simulink model "StarMac_Model"  (Simulink 7.1)
settings: Solver=FixedStepDiscrete  StartTime=0.0  StopTime=10.0  RelTol=1e-3
undefined symbols (not defined in the file or in its folder): schedule, ToverTh
libraries: simulink x10, truetime x2, aero_sim_lib x1
settings Model: Creator=jporter  LastModifiedBy=jporter

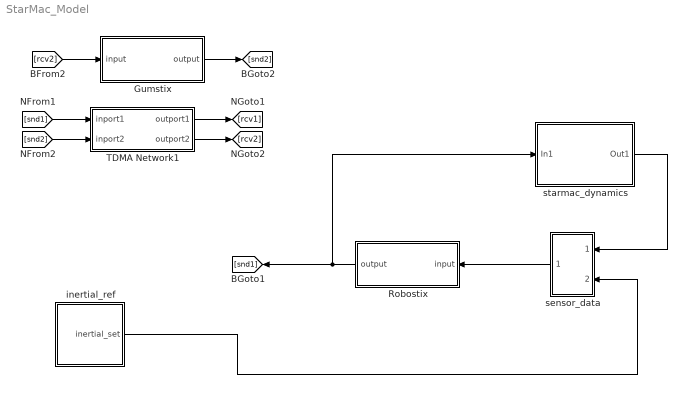
== system StarMac_Model ==
  Gumstix : Subsystem
  Robostix : Subsystem  Orientation=left
  TDMA Network1 : Subsystem
  inertial_ref : Subsystem
  sensor_data : Subsystem  Orientation=left
  starmac_dynamics : Subsystem
  wires:
  inertial_ref/1(inertial_set) -> sensor_data/2(In2)
  starmac_dynamics/1(Out1) -> sensor_data/1(In1)
  TDMA Network1/1(outport1) -> [rcv1]
  [snd1] -> TDMA Network1/1(inport1)
  TDMA Network1/2(outport2) -> [rcv2]
  [snd2] -> TDMA Network1/2(inport2)
  Robostix/1(output) -> [snd1], starmac_dynamics/1(In1)
  [rcv2] -> Gumstix/1(input)
  Gumstix/1(output) -> [snd2]
  sensor_data/1(Out1) -> Robostix/1(input)

== system StarMac_Model/Gumstix ==
  input : Inport
  Ground1 : Ground
  Gumstix_Output : Scope
      settings: DataFormat=Array
  Gumstix_Schedule : Scope
      settings: DataFormat=Array
  Terminator1 : Terminator
  Terminator2 : Terminator
  Terminator3 : Terminator
  TrueTime Kernel : Subsystem  mask{sfun=Generic_Init, args=schedule, clockdrift=0, clockoffset=0}
      mask prompts: sfun "Name of init function (MEX or MATLAB)"; args "Init function argument"; clockdrift "Clock drift"; clockoffset "Clock offset"
  output : Outport
  wires:
  input/1 -> TrueTime Kernel/3(Rcv)
  Ground1/1 -> TrueTime Kernel/1(A/D), TrueTime Kernel/2(Interrupts)
  TrueTime Kernel/2(Snd) -> output/1, Gumstix_Output/1
  TrueTime Kernel/1(D/A) -> Terminator1/1
  TrueTime Kernel/3(Schedule) -> Gumstix_Schedule/1
  TrueTime Kernel/4(Monitors) -> Terminator2/1
  TrueTime Kernel/5(P) -> Terminator3/1

== system StarMac_Model/Robostix ==
  input : Inport
  Ground1 : Ground
  Robostix_Output : Scope
      settings: DataFormat=Array
  Robostix_Schedule : Scope
      settings: DataFormat=Array
  Terminator1 : Terminator
  Terminator2 : Terminator
  Terminator3 : Terminator
  TrueTime Kernel : Subsystem  mask{sfun=Generic_Init, args=schedule, clockdrift=0, clockoffset=0}
      mask prompts: sfun "Name of init function (MEX or MATLAB)"; args "Init function argument"; clockdrift "Clock drift"; clockoffset "Clock offset"
  output : Outport
  wires:
  input/1 -> TrueTime Kernel/3(Rcv)
  Ground1/1 -> TrueTime Kernel/1(A/D), TrueTime Kernel/2(Interrupts)
  TrueTime Kernel/2(Snd) -> output/1, Robostix_Output/1
  TrueTime Kernel/1(D/A) -> Terminator1/1
  TrueTime Kernel/3(Schedule) -> Robostix_Schedule/1
  TrueTime Kernel/4(Monitors) -> Terminator2/1
  TrueTime Kernel/5(P) -> Terminator3/1

== system StarMac_Model/TDMA Network1 ==
  inport1 : Inport
  inport2 : Inport  Port=2
  Demux1 : Demux  Outputs=2
  Mux1 : Mux  Inputs=2
  Network_Schedule : Scope
      settings: DataFormat=Array
  TrueTime Network : Subsystem  mask{nwtype=TDMA, nwnbr=1, nnodes=2, rate=100000, minsize=4096, lossprob=0, bandwidths=[0.5 0.5], slotsize=4096, schedule=[1 2], memsize=671088640, buftype=Common Buffer, overflow=Retransmit}
      mask prompts: nwtype "Network type"; nwnbr "Network number"; nnodes "Number of nodes"; rate "Data rate (bits/s)"; minsize "Minimum frame size (bits)"; lossprob "Loss probability (0-1)"; bandwidths "Bandwidth allocations"; slotsize "Slotsize (bits)"; schedule "Cyclic schedule"; memsize "Total switch memory (bits)"; buftype "Switch buffer type"; overflow "Switch overflow behavior"
      mask StyleString: popup(CSMA/CD (Ethernet)|CSMA/AMP (CAN)|Round Robin|FDMA|TDMA|Switched Ethernet),edit,edit,edit,edit,edit,edit,edit,edit,edit,popup(Common buffer|Symmetric output buffers),popup(Retransmit|Drop)
  outport1 : Outport
  outport2 : Outport  Port=2
  wires:
  Mux1/1 -> TrueTime Network/1(Snd)
  TrueTime Network/1(Rcv) -> Demux1/1
  TrueTime Network/2(Schedule) -> Network_Schedule/1
  Demux1/1 -> outport1/1
  inport1/1 -> Mux1/1
  Demux1/2 -> outport2/1
  inport2/1 -> Mux1/2

== system StarMac_Model/inertial_ref ==
  Signal Generator : SignalGenerator  Amplitude=20*[1 -1 .5]  Frequency=.5*.0625*ones(3,1)
  inertial_set : Outport
  wires:
  Signal Generator/1 -> inertial_set/1

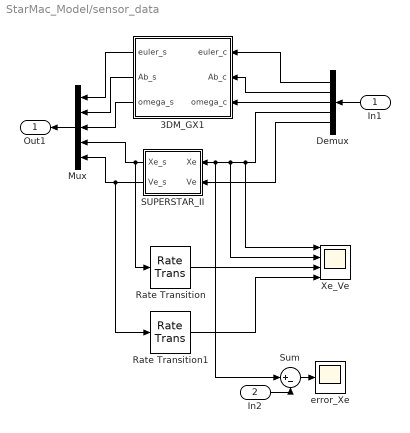
== system StarMac_Model/sensor_data ==
  In1 : Inport  Orientation=left
  In2 : Inport  Port=2
  3DM_GX1 : Subsystem  Orientation=left  mask{a_g_s=7000, g_max=5, g_g_s=8500, omega_max=300, Ts=.01}
      mask prompts: a_g_s "AccelGainScale:"; g_max "Max G (1 G = 9.81 m/s^2):"; g_g_s "GyroGainScale:"; omega_max "Mav Angular Velocity (deg/sec):"; Ts "Sample Rate (seconds):"
  Demux : Demux  Orientation=left  Outputs=5
  Mux : Mux  Orientation=left  Inputs=5
  Rate Transition : RateTransition
  Rate Transition1 : RateTransition
  SUPERSTAR_II : Subsystem  Orientation=left  mask{Ts=.2}
      mask prompts: Ts "Sample Rate (seconds):"
  Sum : Sum  Inputs=|+-  OutDataType=sfix(16)  OutScaling=2^0
  Xe_Ve : Scope  NumInputPorts=4
      settings: YMin=-5~-5~-5~-5  YMax=5~5~5~5
  error_Xe : Scope
  Out1 : Outport  Orientation=left
  wires:
  3DM_GX1/1(euler_s) -> Mux/1
  3DM_GX1/2(Ab_s) -> Mux/2
  3DM_GX1/3(omega_s) -> Mux/3
  SUPERSTAR_II/1(Xe_s) -> Mux/4, Rate Transition/1
  SUPERSTAR_II/2(Ve_s) -> Mux/5, Rate Transition1/1
  Demux/1 -> 3DM_GX1/1(euler_c)
  Demux/2 -> 3DM_GX1/2(Ab_c)
  Demux/3 -> 3DM_GX1/3(omega_c)
  Demux/4 -> Xe_Ve/1, Xe_Ve/2, SUPERSTAR_II/1(Xe), Sum/1
  Demux/5 -> SUPERSTAR_II/2(Ve)
  Rate Transition/1 -> Xe_Ve/3
  Rate Transition1/1 -> Xe_Ve/4
  Sum/1 -> error_Xe/1
  In1/1 -> Demux/1
  Mux/1 -> Out1/1
  In2/1 -> Sum/2

== system StarMac_Model/starmac_dynamics ==
  In1 : Inport
  Mux : Mux  Inputs=5
  Terminator : Terminator
  Terminator1 : Terminator
  starmac_dynamics : Subsystem  AncestorBlock=aero_sim_lib/starmac_dynamics  mask{M=1.8263, tau_motor=0.1, b=0.1, select_sub=Select Subsystem}
      mask prompts: M "UAV Mass (kg) [M]:"; tau_motor "Motor Time constant (s)[tau_motor]:"; b "Viscus Drag Coef. (N-s/m)[b]:"; select_sub "Select a model Subsystem:"
      mask StyleString: edit,edit,edit,popup(Select Subsystem|M:starmac_motor_dynamics|B:starmac_blade_flapping_effects|6:6DOF_Euler_Angles)
      mask CallbackString:
      | |||gcb_d=gcb;
      | mask_str = get_param(gcb_d, 'MaskValues');
      | if strcmp(mask_str{4}(1),'M')
      |     open_system([gcb_d '/starmac_motor_dynamics'],'mask');
      | elseif strcmp(mask_str{4}(1),'B')
      |     open_system([gcb_d '/starmac_blade_flapping_effects'],'mask');
      | elseif strcmp(mask_str{4}(1),'6')
      |     open_system([gcb_d '/6DOF_Euler_Angles'],'mask');
      | else
      |     return
      | end
      | set_param(gcb_d,'select_sub','Select Subsystem');
  wind_velocity : Constant  Value=zeros(3,1)  OutDataType=sfix(16)  OutScaling=2^0
  Out1 : Outport
  wires:
  wind_velocity/1 -> starmac_dynamics/2(wind_velocity)
  starmac_dynamics/1(Ve) -> Mux/1
  starmac_dynamics/2(Xe) -> Mux/2
  starmac_dynamics/4(DCM) -> Terminator/1
  starmac_dynamics/6(domega/dt) -> Terminator1/1
  Mux/1 -> Out1/1
  In1/1 -> starmac_dynamics/1(desired_motor_thrust)
  starmac_dynamics/3(euler) -> Mux/3
  starmac_dynamics/5(omega) -> Mux/4
  starmac_dynamics/7(Ab) -> Mux/5

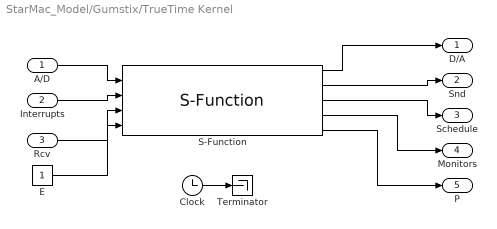
== system StarMac_Model/Gumstix/TrueTime Kernel ==
  A/D : Inport
  Interrupts : Inport  Port=2
  Rcv : Inport  Port=3
  Clock : Clock
      settings: Decimation=10
  E : Constant
  S-Function : truetime/TrueTime Kernel/S-Function
  Terminator : Terminator
  D/A : Outport
  Snd : Outport  Port=2
  Schedule : Outport  Port=3
  Monitors : Outport  Port=4
  P : Outport  Port=5
  wires:
  S-Function/5 -> P/1
  E/1 -> S-Function/4
  A/D/1 -> S-Function/1
  S-Function/2 -> Snd/1
  S-Function/1 -> D/A/1
  S-Function/3 -> Schedule/1
  S-Function/4 -> Monitors/1
  Interrupts/1 -> S-Function/2
  Rcv/1 -> S-Function/3
  Clock/1 -> Terminator/1

== system StarMac_Model/Robostix/TrueTime Kernel ==
  A/D : Inport
  Interrupts : Inport  Port=2
  Rcv : Inport  Port=3
  Clock : Clock
      settings: Decimation=10
  E : Constant
  S-Function : truetime/TrueTime Kernel/S-Function
  Terminator : Terminator
  D/A : Outport
  Snd : Outport  Port=2
  Schedule : Outport  Port=3
  Monitors : Outport  Port=4
  P : Outport  Port=5
  wires:
  S-Function/5 -> P/1
  E/1 -> S-Function/4
  A/D/1 -> S-Function/1
  S-Function/2 -> Snd/1
  S-Function/1 -> D/A/1
  S-Function/3 -> Schedule/1
  S-Function/4 -> Monitors/1
  Interrupts/1 -> S-Function/2
  Rcv/1 -> S-Function/3
  Clock/1 -> Terminator/1

== system StarMac_Model/TDMA Network1/TrueTime Network ==
  Snd : Inport
  ttnetwork : S-Function  FunctionName=ttnetwork  Parameters=nwtype,nwnbr,nnodes,rate,minsize,lossprob,bandwidths,slotsize,schedule,memsize,buftype,overflow  EnableBusSupport=off
  Rcv : Outport
  Schedule : Outport  Port=2
  wires:
  ttnetwork/2 -> Schedule/1
  ttnetwork/1 -> Rcv/1
  Snd/1 -> ttnetwork/1

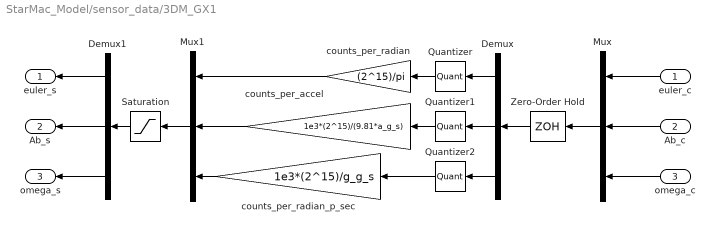
== system StarMac_Model/sensor_data/3DM_GX1 ==
  euler_c : Inport  Orientation=left
  Ab_c : Inport  Orientation=left  Port=2
  omega_c : Inport  Orientation=left  Port=3
  Demux : Demux  Orientation=left  Outputs=[3 3 3]
  Demux1 : Demux  Orientation=left  Outputs=[3 3 3]
  Mux : Mux  Orientation=left  Inputs=[3 3 3]
  Mux1 : Mux  Orientation=left  Inputs=3
  Quantizer : Quantizer  Orientation=left  QuantizationInterval=pi/(2^15)*ones(3,1)
  Quantizer1 : Quantizer  Orientation=left  QuantizationInterval=g_max*9.81/(2^15)*ones(3,1)
  Quantizer2 : Quantizer  Orientation=left  QuantizationInterval=(pi*omega_max/180)/(2^15)*ones(3,1)
  Saturation : Saturate  Orientation=left  UpperLimit=((2^15)-1)*ones(3*3,1)  LowerLimit=-(2^15)*ones(3*3,1)  OutDataType=sfix(16)  OutScaling=2^0
  Zero-Order Hold : ZeroOrderHold  Orientation=left  SampleTime=Ts
  counts_per_accel : Gain  Orientation=left  Gain=1e3*(2^15)/(9.81*a_g_s)  ParameterDataType=sfix(16)  ParameterScaling=2^0  OutDataType=sfix(16)  OutScaling=2^0
  counts_per_radian : Gain  Orientation=left  Gain=(2^15)/pi  ParameterDataType=sfix(16)  ParameterScaling=2^0  OutDataType=sfix(16)  OutScaling=2^0
  counts_per_radian_p_sec : Gain  Orientation=left  Gain=1e3*(2^15)/g_g_s  ParameterDataType=sfix(16)  ParameterScaling=2^0  OutDataType=sfix(16)  OutScaling=2^0
  euler_s : Outport  Orientation=left
  Ab_s : Outport  Orientation=left  Port=2
  omega_s : Outport  Orientation=left  Port=3
  wires:
  Mux/1 -> Zero-Order Hold/1
  euler_c/1 -> Mux/1
  Ab_c/1 -> Mux/2
  omega_c/1 -> Mux/3
  Zero-Order Hold/1 -> Demux/1
  Demux/1 -> Quantizer/1
  Demux/2 -> Quantizer1/1
  Quantizer/1 -> counts_per_radian/1
  Quantizer1/1 -> counts_per_accel/1
  counts_per_accel/1 -> Mux1/2
  counts_per_radian/1 -> Mux1/1
  Demux/3 -> Quantizer2/1
  counts_per_radian_p_sec/1 -> Mux1/3
  Quantizer2/1 -> counts_per_radian_p_sec/1
  Mux1/1 -> Saturation/1
  Saturation/1 -> Demux1/1
  Demux1/1 -> euler_s/1
  Demux1/2 -> Ab_s/1
  Demux1/3 -> omega_s/1

== system StarMac_Model/sensor_data/SUPERSTAR_II ==
  Xe : Inport  Orientation=left
  Ve : Inport  Orientation=left  Port=2
  Demux : Demux  Orientation=left  Outputs=[3 3]
  Mux : Mux  Orientation=left  Inputs=[3 3]
  ZOH : ZeroOrderHold  Orientation=left  SampleTime=Ts
  Xe_s : Outport  Orientation=left
  Ve_s : Outport  Orientation=left  Port=2
  wires:
  ZOH/1 -> Demux/1
  Ve/1 -> Mux/2
  Xe/1 -> Mux/1
  Mux/1 -> ZOH/1
  Demux/1 -> Xe_s/1
  Demux/2 -> Ve_s/1

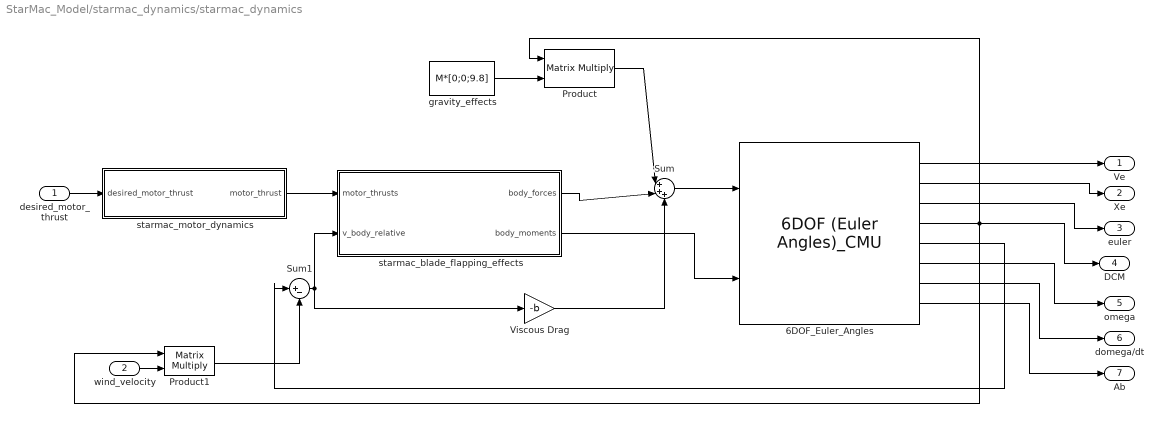
== system StarMac_Model/starmac_dynamics/starmac_dynamics ==
  desired_motor_thrust : Inport  OutDataType=sfix(16)  OutScaling=2^0
  wind_velocity : Inport  Port=2  OutDataType=sfix(16)  OutScaling=2^0
  6DOF_Euler_Angles : aero_sim_lib/6DOF (Euler Angles)_CMU  SystemSampleTime=-1  XYZe_0=[0.1;0.2;0]  Vb_0=[0;0;0]  euler_0=[0;0;0]  omega_0=[0;0;0]  M=M  I=diag([0.02759 0.02771 0.04806])
  Product : Product  Multiplication=Matrix(*)  OutDataType=sfix(16)  OutScaling=2^0  RndMeth=Zero
  Product1 : Product  Multiplication=Matrix(*)  OutDataType=sfix(16)  OutScaling=2^0  RndMeth=Zero
  Sum : Sum  Inputs=|+++  OutDataType=sfix(16)  OutScaling=2^0
  Sum1 : Sum  Inputs=|+-  OutDataType=sfix(16)  OutScaling=2^0
  Viscous Drag : Gain  Gain=-b  ParameterDataType=sfix(16)  ParameterScaling=2^0  OutDataType=sfix(16)  OutScaling=2^0
  gravity_effects : Constant  Value=M*[0;0;9.8]  OutDataType=sfix(16)  OutScaling=2^0
  starmac_blade_flapping_effects : Subsystem  AncestorBlock=aero_sim_lib/starmac_blade_flapping_effects  mask{select_sub=Select Subsystem}
      mask prompts: select_sub "Select Subsystem:"
      mask help:
      | Allows user to set parameters of various subsystems
      | within the Blade Flapping Effects Model
      mask Help:
      | Select a Subsystem To Set Various
      | Sub System Parameters
      mask StyleString: popup(Select Subsystem|V:starmac_vertical_effect_dynamics|B:starmac_body_moments|F:starmac_flapping_dynamics)
      mask CallbackString:
      | gcb_c=gcb;
      | mask_str = get_param(gcb_c, 'MaskValues');
      | if strcmp(mask_str{1}(1),'V')
      |     open_system([gcb_c '/starmac_vertical_effect_dynamics'],'mask');
      | elseif strcmp(mask_str{1}(1),'B')
      |     open_system([gcb_c '/starmac_body_moments'],'mask');
      | elseif strcmp(mask_str{1}(1),'F')
      |     open_system([gcb_c '/starmac_flapping_dynamics'],'mask');
      | else
      |     return
      | end
      | set_param(gcb_c,'select_sub','Select Subsystem');
  starmac_motor_dynamics : Subsystem  AncestorBlock=aero_sim_lib/starmac_motor_dynamics  mask{tau_motor=tau_motor, T_nom=M*9.8/4, thrust_max=9.8, thrust_min=0, motor_lag_enable=on, motor_variance=(.05*9.8/4)^2, Ts=.01}
      mask prompts: tau_motor "tau_motor (seconds):"; T_nom "nominal thrust (N):"; thrust_max "maximum thrust (N):"; thrust_min "minimum thrust (N):"; motor_lag_enable "Motor Lag Enabled:"; motor_variance "Motor Variance [motor_variance]:"; Ts "Motor Update Rate (seconds):"
  Ve : Outport  OutDataType=sfix(16)  OutScaling=2^0
  Xe : Outport  Port=2  OutDataType=sfix(16)  OutScaling=2^0
  euler : Outport  Port=3  OutDataType=sfix(16)  OutScaling=2^0
  DCM : Outport  Port=4  OutDataType=sfix(16)  OutScaling=2^0
  omega : Outport  Port=5  OutDataType=sfix(16)  OutScaling=2^0
  domega/dt : Outport  Port=6  OutDataType=sfix(16)  OutScaling=2^0
  Ab : Outport  Port=7  OutDataType=sfix(16)  OutScaling=2^0
  wires:
  6DOF_Euler_Angles/8 -> Ab/1
  6DOF_Euler_Angles/7 -> domega/dt/1
  6DOF_Euler_Angles/6 -> omega/1
  6DOF_Euler_Angles/3 -> euler/1
  6DOF_Euler_Angles/2 -> Xe/1
  6DOF_Euler_Angles/1 -> Ve/1
  starmac_motor_dynamics/1(motor_thrust) -> starmac_blade_flapping_effects/1(motor_thrusts)
  Product/1 -> Sum/1
  Sum/1 -> 6DOF_Euler_Angles/1
  6DOF_Euler_Angles/4 -> DCM/1, Product/1, Product1/1
  gravity_effects/1 -> Product/2
  Sum1/1 -> starmac_blade_flapping_effects/2(v_body_relative), Viscous Drag/1
  Product1/1 -> Sum1/2
  6DOF_Euler_Angles/5 -> Sum1/1
  Viscous Drag/1 -> Sum/3
  starmac_blade_flapping_effects/2(body_moments) -> 6DOF_Euler_Angles/2
  starmac_blade_flapping_effects/1(body_forces) -> Sum/2
  desired_motor_thrust/1 -> starmac_motor_dynamics/1(desired_motor_thrust)
  wind_velocity/1 -> Product1/2

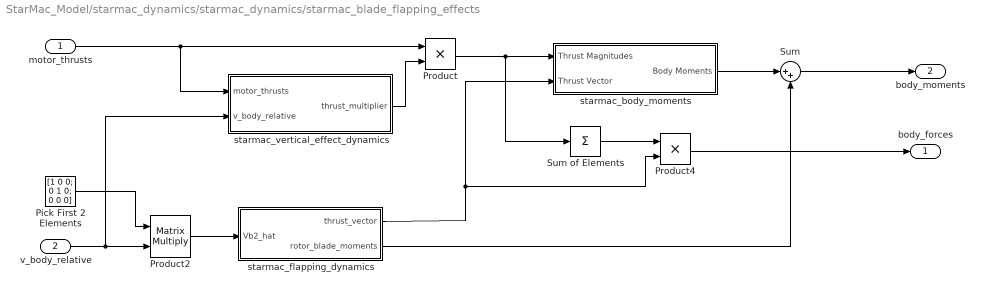
== system StarMac_Model/starmac_dynamics/starmac_dynamics/starmac_blade_flapping_effects ==
  motor_thrusts : Inport  OutDataType=sfix(16)  OutScaling=2^0
  v_body_relative : Inport  Port=2  OutDataType=sfix(16)  OutScaling=2^0
  Pick First 2 Elements : Constant  Value=[1 0 0; 0 1 0; 0 0 0]  OutDataType=sfix(16)  OutScaling=2^0
  Product : Product  OutDataType=sfix(16)  OutScaling=2^0  RndMeth=Zero
  Product2 : Product  Multiplication=Matrix(*)  OutDataType=sfix(16)  OutScaling=2^0  RndMeth=Zero
  Product4 : Product  OutDataType=sfix(16)  OutScaling=2^0  RndMeth=Zero
  Sum : Sum  Inputs=|++  OutDataType=sfix(16)  OutScaling=2^0
  Sum of Elements : Sum  Inputs=+  OutDataType=sfix(16)  OutScaling=2^-10
  starmac_body_moments : Subsystem  AncestorBlock=aero_sim_lib/starmac_body_moments  mask{dx=.3048, dz=.07, K_torque=.47}
  starmac_flapping_dynamics : Subsystem  AncestorBlock=aero_sim_lib/starmac_flapping_dynamics  mask{K_a1s=.009, K_beta=.23}
  starmac_vertical_effect_dynamics : Subsystem  AncestorBlock=aero_sim_lib/starmac_vertical_effect_dynamics  mask{tau_motor=tau_motor, R=0.127, Alpha=(pi/180)*[-85:5:85], Vinf=[0:0.5:6], Thrust=9.8*[0.3:0.02:0.8]}
      mask prompts: tau_motor "motor time constant (s)"; R "radius of propeller (m)"; Alpha "Alpha (radians)"; Vinf "Vinf (radians)"; Thrust "Propeller Thrust (N)"
      mask init:
      | rho = 1.2;
      | A = pi*R^2;
      | Vh = sqrt(Thrust/(2*rho*A));
      | for i = 1:length(Vh)
      |     for j = 1:length(Vinf)
      |         for k = 1:length(Alpha)
      |             Vi(k,j,i) = find_vi(Vh(i),Vinf(j),Alpha(k));
      |             ToverTh(k,j,i) = min(10,max(0.1,Vh(i)/(Vi(k,j,i)+Vinf(j)*sin(Alpha(k)))));
      |         end
      |     end
      | end
  body_forces : Outport  OutDataType=sfix(16)  OutScaling=2^0
  body_moments : Outport  Port=2  OutDataType=sfix(16)  OutScaling=2^0
  wires:
  starmac_flapping_dynamics/2(rotor_blade_moments) -> Sum/2
  Sum/1 -> body_moments/1
  starmac_body_moments/1(Body Moments) -> Sum/1
  starmac_flapping_dynamics/1(thrust_vector) -> Product4/2, starmac_body_moments/2(Thrust Vector)
  Product4/1 -> body_forces/1
  Sum of Elements/1 -> Product4/1
  Product2/1 -> starmac_flapping_dynamics/1(Vb2_hat)
  v_body_relative/1 -> Product2/2, starmac_vertical_effect_dynamics/2(v_body_relative)
  Pick First 2 Elements/1 -> Product2/1
  motor_thrusts/1 -> Product/1, starmac_vertical_effect_dynamics/1(motor_thrusts)
  starmac_vertical_effect_dynamics/1(thrust_multiplier) -> Product/2
  Product/1 -> Sum of Elements/1, starmac_body_moments/1(Thrust Magnitudes)

== system StarMac_Model/starmac_dynamics/starmac_dynamics/starmac_motor_dynamics ==
  desired_motor_thrust : Inport  OutDataType=sfix(16)  OutScaling=2^0
  Band-Limited White Noise : simulink/Sources/Band-Limited White Noise  SystemSampleTime=-1  Cov=Ts*motor_variance*ones(4,1)  Ts=Ts  seed=22341+[0 1 2 3]'
  Constant : Constant  Value=motor_lag_enable  OutDataType=sfix(16)  OutScaling=2^0
  Rate Transition : RateTransition
  Saturation : Saturate  UpperLimit=thrust_max*ones(4,1)  LowerLimit=thrust_min*ones(4,1)
  State-Space : StateSpace  A=-(1/tau_motor)*eye(4)  B=(1/tau_motor)*eye(4)  C=eye(4)  D=zeros(4,4)  X0=T_nom*ones(4,1)
  Sum : Sum  Inputs=|++  OutDataType=sfix(16)  OutScaling=2^0
  Switch : Switch  Criteria=u2 > Threshold  OutDataType=sfix(16)  OutScaling=2^0
  motor_thrust : Outport  OutDataType=sfix(16)  OutScaling=2^0
  wires:
  desired_motor_thrust/1 -> State-Space/1, Switch/3
  Sum/1 -> motor_thrust/1
  Saturation/1 -> Sum/1
  Band-Limited White Noise/1 -> Rate Transition/1
  State-Space/1 -> Switch/1
  Switch/1 -> Saturation/1
  Constant/1 -> Switch/2
  Rate Transition/1 -> Sum/2

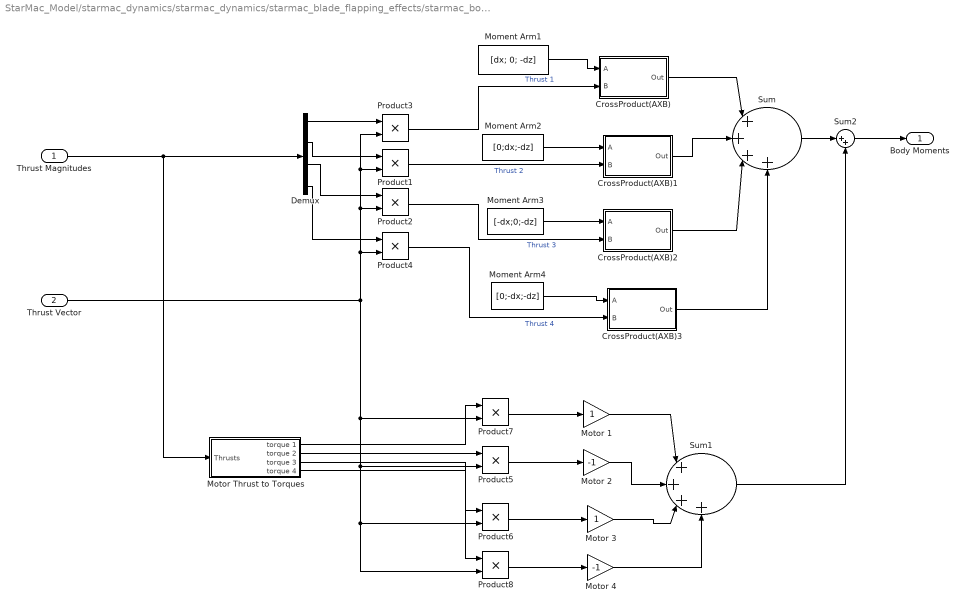
== system StarMac_Model/starmac_dynamics/starmac_dynamics/starmac_blade_flapping_effects/starmac_body_moments ==
  Thrust Magnitudes : Inport  OutDataType=sfix(16)  OutScaling=2^0
  Thrust Vector : Inport  Port=2  OutDataType=sfix(16)  OutScaling=2^0
  CrossProduct(AXB) : Subsystem
  CrossProduct(AXB)1 : Subsystem
  CrossProduct(AXB)2 : Subsystem
  CrossProduct(AXB)3 : Subsystem
  Demux : Demux
  Moment Arm1 : Constant  Value=[dx; 0; -dz]  OutDataType=sfix(16)  OutScaling=2^0
  Moment Arm2 : Constant  Value=[0;dx;-dz]  OutDataType=sfix(16)  OutScaling=2^0
  Moment Arm3 : Constant  Value=[-dx;0;-dz]  OutDataType=sfix(16)  OutScaling=2^0
  Moment Arm4 : Constant  Value=[0;-dx;-dz]  OutDataType=sfix(16)  OutScaling=2^0
  Motor 1 : Gain  ParameterDataType=sfix(16)  ParameterScaling=2^0  OutDataType=sfix(16)  OutScaling=2^0
  Motor 2 : Gain  Gain=-1  ParameterDataType=sfix(16)  ParameterScaling=2^0  OutDataType=sfix(16)  OutScaling=2^0
  Motor 3 : Gain  ParameterDataType=sfix(16)  ParameterScaling=2^0  OutDataType=sfix(16)  OutScaling=2^0
  Motor 4 : Gain  Gain=-1  ParameterDataType=sfix(16)  ParameterScaling=2^0  OutDataType=sfix(16)  OutScaling=2^0
  Motor Thrust to Torques : Subsystem
  Product{1..8} (8 alike) : Product  OutDataType=sfix(16)  OutScaling=2^0  RndMeth=Zero
  Sum : Sum  Inputs=|++++  OutDataType=sfix(16)  OutScaling=2^0
  Sum1 : Sum  Inputs=|++++  OutDataType=sfix(16)  OutScaling=2^0
  Sum2 : Sum  Inputs=|++  OutDataType=sfix(16)  OutScaling=2^0
  Body Moments : Outport  OutDataType=sfix(16)  OutScaling=2^0
  wires:
  CrossProduct(AXB)1/1(Out) -> Sum/2
  Motor Thrust to Torques/4(torque 4) -> Product8/1
  Motor Thrust to Torques/3(torque 3) -> Product6/1
  Motor Thrust to Torques/2(torque 2) -> Product5/1
  Motor Thrust to Torques/1(torque 1) -> Product7/1
  Product8/1 -> Motor 4/1
  Product6/1 -> Motor 3/1
  Product5/1 -> Motor 2/1
  Product7/1 -> Motor 1/1
  Sum2/1 -> Body Moments/1
  Sum1/1 -> Sum2/2
  Sum/1 -> Sum2/1
  Motor 4/1 -> Sum1/4
  Motor 3/1 -> Sum1/3
  Motor 2/1 -> Sum1/2
  Motor 1/1 -> Sum1/1
  CrossProduct(AXB)3/1(Out) -> Sum/4
  CrossProduct(AXB)2/1(Out) -> Sum/3
  CrossProduct(AXB)/1(Out) -> Sum/1
  Product4/1 -> CrossProduct(AXB)3/2(B)  "Thrust 4"
  Moment Arm4/1 -> CrossProduct(AXB)3/1(A)
  Product2/1 -> CrossProduct(AXB)2/2(B)  "Thrust 3"
  Moment Arm3/1 -> CrossProduct(AXB)2/1(A)
  Product1/1 -> CrossProduct(AXB)1/2(B)  "Thrust 2"
  Moment Arm2/1 -> CrossProduct(AXB)1/1(A)
  Product3/1 -> CrossProduct(AXB)/2(B)  "Thrust 1"
  Moment Arm1/1 -> CrossProduct(AXB)/1(A)
  Thrust Vector/1 -> Product8/2, Product6/2, Product5/2, Product7/2, Product4/2, Product2/2, Product1/2, Product3/2
  Demux/4 -> Product4/1
  Demux/3 -> Product2/1
  Demux/2 -> Product1/1
  Demux/1 -> Product3/1
  Thrust Magnitudes/1 -> Motor Thrust to Torques/1(Thrusts), Demux/1

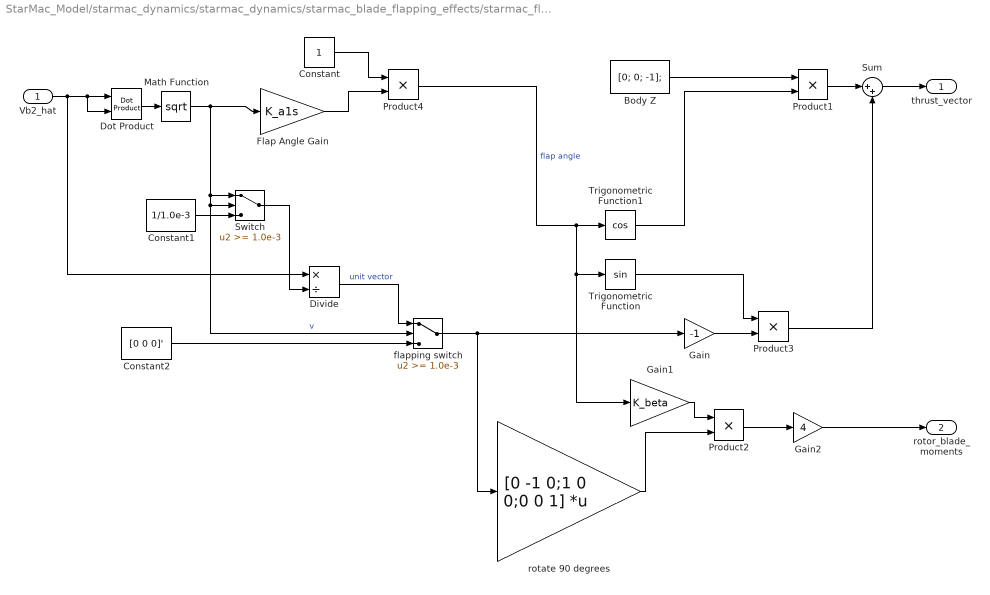
== system StarMac_Model/starmac_dynamics/starmac_dynamics/starmac_blade_flapping_effects/starmac_flapping_dynamics ==
  Vb2_hat : Inport  OutDataType=sfix(16)  OutScaling=2^0
  "Body Z " : Constant  Value=[0; 0; -1];  OutDataType=sfix(16)  OutScaling=2^0
  Constant : Constant  OutDataType=sfix(16)  OutScaling=2^0
  Constant1 : Constant  Value=1/1.0e-3  OutDataType=sfix(16)  OutScaling=2^0
  Constant2 : Constant  Value=[0 0 0]'  OutDataType=sfix(16)  OutScaling=2^0
  Divide : Product  Inputs=*/  OutDataType=sfix(16)  OutScaling=2^-10
  Dot Product : simulink/Math Operations/Dot Product  InputSameDT=on  OutDataType=sfix(16)  OutScaling=2^-10  DoSatur=off
  Flap Angle Gain : Gain  Gain=K_a1s  ParameterDataType=sfix(16)  ParameterScaling=2^0  OutDataType=sfix(16)  OutScaling=2^0
  Gain : Gain  Gain=-1  ParameterDataType=sfix(16)  ParameterScaling=2^0  OutDataType=sfix(16)  OutScaling=2^0
  Gain1 : Gain  Gain=K_beta  ParameterDataType=sfix(16)  ParameterScaling=2^0  OutDataType=sfix(16)  OutScaling=2^0
  Gain2 : Gain  Gain=4  ParameterDataType=sfix(16)  ParameterScaling=2^0  OutDataType=sfix(16)  OutScaling=2^0
  Math Function : Math  Operator=sqrt  OutDataType=sfix(16)  OutScaling=2^0  SaturateOnIntegerOverflow=on
  Product{1..4} (4 alike) : Product  OutDataType=sfix(16)  OutScaling=2^0  RndMeth=Zero
  Sum : Sum  Inputs=|++  OutDataType=sfix(16)  OutScaling=2^0
  Switch : Switch  Threshold=1.0e-3
  Trigonometric Function : Trigonometry
  Trigonometric Function1 : Trigonometry  Operator=cos
  flapping switch : Switch  Threshold=1.0e-3
  rotate 90 degrees : Gain  Gain=[0 -1 0;1 0 0;0 0 1]  Multiplication=Matrix(K*u)  ParameterDataType=sfix(16)  ParameterScaling=2^0  OutDataType=sfix(16)  OutScaling=2^0
  thrust_vector : Outport  OutDataType=sfix(16)  OutScaling=2^0
  rotor_blade_moments : Outport  Port=2  OutDataType=sfix(16)  OutScaling=2^0
  wires:
  Constant/1 -> Product4/1
  Flap Angle Gain/1 -> Product4/2
  Gain1/1 -> Product2/1
  rotate 90 degrees/1 -> Product2/2
  Product2/1 -> Gain2/1
  Constant2/1 -> flapping switch/3
  flapping switch/1 -> rotate 90 degrees/1, Gain/1
  Divide/1 -> flapping switch/1  "unit vector"
  Constant1/1 -> Switch/3
  Switch/1 -> Divide/2
  Gain2/1 -> rotor_blade_moments/1
  Sum/1 -> thrust_vector/1
  "Body Z "/1 -> Product1/1
  Product1/1 -> Sum/1
  Gain/1 -> Product3/2
  Product3/1 -> Sum/2
  Trigonometric Function/1 -> Product3/1
  Trigonometric Function1/1 -> Product1/2
  Math Function/1 -> Flap Angle Gain/1, flapping switch/2, Switch/2, Switch/1  "v"
  Dot Product/1 -> Math Function/1
  Vb2_hat/1 -> Divide/1, Dot Product/2, Dot Product/1
  Product4/1 -> Gain1/1, Trigonometric Function/1, Trigonometric Function1/1  "flap angle"

== system StarMac_Model/starmac_dynamics/starmac_dynamics/starmac_blade_flapping_effects/starmac_vertical_effect_dynamics ==
  motor_thrusts : Inport  OutDataType=sfix(16)  OutScaling=2^0
  v_body_relative : Inport  Port=2  OutDataType=sfix(16)  OutScaling=2^0
  Demux : Demux
  Mux : Mux
  starmac_motor_vertical_effect_dynamics : Subsystem  AncestorBlock=aero_sim_lib/starmac_motor_vertical_effect_dynamics  mask{tau_motor=tau_motor, R=R, Alpha=Alpha, Vinf=Vinf, Vh=Vh, ToverTh=ToverTh}
      mask prompts: tau_motor "motor time constant (s)"; R "radius of propeller (m)"; Alpha "Alpha (radians):"; Vinf "Vinf (m/s):"; Vh "Vh (m/s):"
      mask init:
      | rho=1.2;    % kg/m^3, density of air
      | A = pi*R^2; % m^2, area swept out by 1 rotor
  starmac_motor_vertical_effect_dynamics1 : Subsystem  AncestorBlock=aero_sim_lib/starmac_motor_vertical_effect_dynamics  mask{tau_motor=tau_motor, R=R, Alpha=Alpha, Vinf=Vinf, Vh=Vh, ToverTh=ToverTh}
      mask prompts: tau_motor "motor time constant (s)"; R "radius of propeller (m)"; Alpha "Alpha (radians):"; Vinf "Vinf (m/s):"; Vh "Vh (m/s):"
      mask init:
      | rho=1.2;    % kg/m^3, density of air
      | A = pi*R^2; % m^2, area swept out by 1 rotor
  starmac_motor_vertical_effect_dynamics2 : Subsystem  AncestorBlock=aero_sim_lib/starmac_motor_vertical_effect_dynamics  mask{tau_motor=tau_motor, R=R, Alpha=Alpha, Vinf=Vinf, Vh=Vh, ToverTh=ToverTh}
      mask prompts: tau_motor "motor time constant (s)"; R "radius of propeller (m)"; Alpha "Alpha (radians):"; Vinf "Vinf (m/s):"; Vh "Vh (m/s):"
      mask init:
      | rho=1.2;    % kg/m^3, density of air
      | A = pi*R^2; % m^2, area swept out by 1 rotor
  starmac_motor_vertical_effect_dynamics3 : Subsystem  AncestorBlock=aero_sim_lib/starmac_motor_vertical_effect_dynamics  mask{tau_motor=tau_motor, R=R, Alpha=Alpha, Vinf=Vinf, Vh=Vh, ToverTh=ToverTh}
      mask prompts: tau_motor "motor time constant (s)"; R "radius of propeller (m)"; Alpha "Alpha (radians):"; Vinf "Vinf (m/s):"; Vh "Vh (m/s):"
      mask init:
      | rho=1.2;    % kg/m^3, density of air
      | A = pi*R^2; % m^2, area swept out by 1 rotor
  thrust_multiplier : Outport  OutDataType=sfix(16)  OutScaling=2^0
  wires:
  motor_thrusts/1 -> Demux/1
  Mux/1 -> thrust_multiplier/1
  Demux/1 -> starmac_motor_vertical_effect_dynamics/1(motor_thrusts)
  Demux/2 -> starmac_motor_vertical_effect_dynamics1/1(motor_thrusts)
  Demux/3 -> starmac_motor_vertical_effect_dynamics2/1(motor_thrusts)
  Demux/4 -> starmac_motor_vertical_effect_dynamics3/1(motor_thrusts)
  starmac_motor_vertical_effect_dynamics/1(thrust_multiplier) -> Mux/1
  starmac_motor_vertical_effect_dynamics1/1(thrust_multiplier) -> Mux/2
  starmac_motor_vertical_effect_dynamics2/1(thrust_multiplier) -> Mux/3
  starmac_motor_vertical_effect_dynamics3/1(thrust_multiplier) -> Mux/4
  v_body_relative/1 -> starmac_motor_vertical_effect_dynamics2/2(v_body_relative), starmac_motor_vertical_effect_dynamics3/2(v_body_relative), starmac_motor_vertical_effect_dynamics1/2(v_body_relative), starmac_motor_vertical_effect_dynamics/2(v_body_relative)

== system StarMac_Model/starmac_dynamics/starmac_dynamics/starmac_blade_flapping_effects/starmac_body_moments/CrossProduct(AXB) ==
  A : Inport  OutDataType=sfix(16)  OutScaling=2^0
  B : Inport  Port=2  OutDataType=sfix(16)  OutScaling=2^0
  Fcn : Fcn  Expr=u[2]*u[6]-u[3]*u[5]
  Fcn1 : Fcn  Expr=u[3]*u[4]-u[1]*u[6]
  Fcn2 : Fcn  Expr=u[1]*u[5]-u[2]*u[4]
  Mux : Mux  Inputs=2
  Mux1 : Mux  Inputs=3
  Out : Outport  OutDataType=sfix(16)  OutScaling=2^0
  wires:
  Mux1/1 -> Out/1
  Fcn2/1 -> Mux1/3
  Fcn1/1 -> Mux1/2
  Fcn/1 -> Mux1/1
  Mux/1 -> Fcn2/1, Fcn1/1, Fcn/1
  B/1 -> Mux/2
  A/1 -> Mux/1

== system StarMac_Model/starmac_dynamics/starmac_dynamics/starmac_blade_flapping_effects/starmac_body_moments/CrossProduct(AXB)1 ==
  A : Inport  OutDataType=sfix(16)  OutScaling=2^0
  B : Inport  Port=2  OutDataType=sfix(16)  OutScaling=2^0
  Fcn : Fcn  Expr=u[2]*u[6]-u[3]*u[5]
  Fcn1 : Fcn  Expr=u[3]*u[4]-u[1]*u[6]
  Fcn2 : Fcn  Expr=u[1]*u[5]-u[2]*u[4]
  Mux : Mux  Inputs=2
  Mux1 : Mux  Inputs=3
  Out : Outport  OutDataType=sfix(16)  OutScaling=2^0
  wires:
  A/1 -> Mux/1
  B/1 -> Mux/2
  Mux/1 -> Fcn/1, Fcn1/1, Fcn2/1
  Fcn/1 -> Mux1/1
  Fcn1/1 -> Mux1/2
  Fcn2/1 -> Mux1/3
  Mux1/1 -> Out/1

== system StarMac_Model/starmac_dynamics/starmac_dynamics/starmac_blade_flapping_effects/starmac_body_moments/CrossProduct(AXB)2 ==
  A : Inport  OutDataType=sfix(16)  OutScaling=2^0
  B : Inport  Port=2  OutDataType=sfix(16)  OutScaling=2^0
  Fcn : Fcn  Expr=u[2]*u[6]-u[3]*u[5]
  Fcn1 : Fcn  Expr=u[3]*u[4]-u[1]*u[6]
  Fcn2 : Fcn  Expr=u[1]*u[5]-u[2]*u[4]
  Mux : Mux  Inputs=2
  Mux1 : Mux  Inputs=3
  Out : Outport  OutDataType=sfix(16)  OutScaling=2^0
  wires:
  Mux1/1 -> Out/1
  Fcn2/1 -> Mux1/3
  Fcn1/1 -> Mux1/2
  Fcn/1 -> Mux1/1
  Mux/1 -> Fcn2/1, Fcn1/1, Fcn/1
  B/1 -> Mux/2
  A/1 -> Mux/1

== system StarMac_Model/starmac_dynamics/starmac_dynamics/starmac_blade_flapping_effects/starmac_body_moments/CrossProduct(AXB)3 ==
  A : Inport  OutDataType=sfix(16)  OutScaling=2^0
  B : Inport  Port=2  OutDataType=sfix(16)  OutScaling=2^0
  Fcn : Fcn  Expr=u[2]*u[6]-u[3]*u[5]
  Fcn1 : Fcn  Expr=u[3]*u[4]-u[1]*u[6]
  Fcn2 : Fcn  Expr=u[1]*u[5]-u[2]*u[4]
  Mux : Mux  Inputs=2
  Mux1 : Mux  Inputs=3
  Out : Outport  OutDataType=sfix(16)  OutScaling=2^0
  wires:
  A/1 -> Mux/1
  B/1 -> Mux/2
  Mux/1 -> Fcn/1, Fcn1/1, Fcn2/1
  Fcn/1 -> Mux1/1
  Fcn1/1 -> Mux1/2
  Fcn2/1 -> Mux1/3
  Mux1/1 -> Out/1

== system StarMac_Model/starmac_dynamics/starmac_dynamics/starmac_blade_flapping_effects/starmac_body_moments/Motor Thrust to Torques ==
  Thrusts : Inport  OutDataType=sfix(16)  OutScaling=2^0
  Demux : Demux
  Gain1 : Gain  Gain=K_torque  ParameterDataType=sfix(16)  ParameterScaling=2^0  OutDataType=sfix(16)  OutScaling=2^0
  torque 1 : Outport  OutDataType=sfix(16)  OutScaling=2^0
  torque 2 : Outport  Port=2  OutDataType=sfix(16)  OutScaling=2^0
  torque 3 : Outport  Port=3  OutDataType=sfix(16)  OutScaling=2^0
  torque 4 : Outport  Port=4  OutDataType=sfix(16)  OutScaling=2^0
  wires:
  Demux/4 -> torque 4/1
  Demux/3 -> torque 3/1
  Demux/2 -> torque 2/1
  Demux/1 -> torque 1/1
  Gain1/1 -> Demux/1
  Thrusts/1 -> Gain1/1

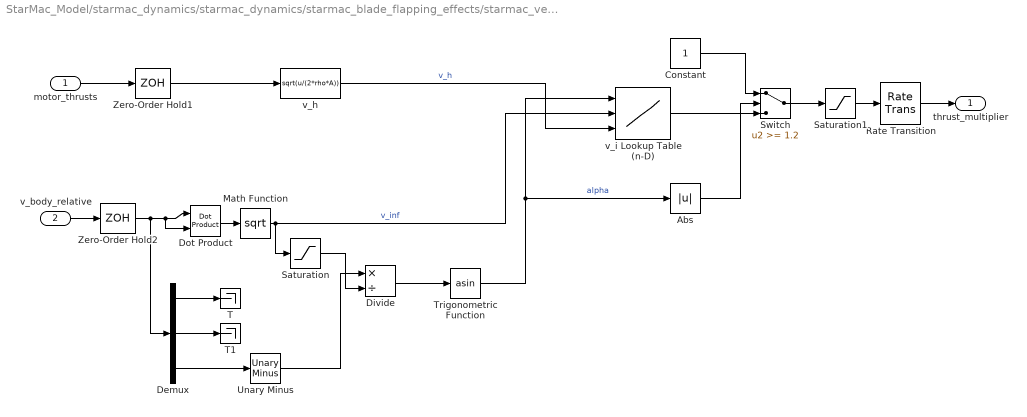
== system StarMac_Model/starmac_dynamics/starmac_dynamics/starmac_blade_flapping_effects/starmac_vertical_effect_dynamics/starmac_motor_vertical_effect_dynamics ==
  motor_thrusts : Inport  OutDataType=sfix(16)  OutScaling=2^0
  v_body_relative : Inport  Port=2  OutDataType=sfix(16)  OutScaling=2^0
  Abs : Abs
  Constant : Constant  OutDataType=sfix(16)  OutScaling=2^0
  Demux : Demux  Outputs=3
  Divide : Product  Inputs=*/  OutDataType=sfix(16)  OutScaling=2^-10
  Dot Product : simulink/Math Operations/Dot Product  InputSameDT=on  OutDataType=sfix(16)  OutScaling=2^-10  DoSatur=off
  Math Function : Math  Operator=sqrt  OutDataType=sfix(16)  OutScaling=2^0  SaturateOnIntegerOverflow=on
  Rate Transition : RateTransition
  Saturation : Saturate  UpperLimit=500000  LowerLimit=0.0000000001
  Saturation1 : Saturate  UpperLimit=2  LowerLimit=0.5
  Switch : Switch  Threshold=1.2
  T : Terminator
  T1 : Terminator
  Trigonometric Function : Trigonometry  Operator=asin
  Unary Minus : simulink/Math Operations/Unary Minus  DoSatur=off
  Zero-Order Hold1 : ZeroOrderHold  SampleTime=tau_motor
  Zero-Order Hold2 : ZeroOrderHold  SampleTime=tau_motor
  "v_h " : Fcn  Expr=sqrt(u/(2*rho*A))
  v_i Lookup Table (n-D) : Lookup_n-D  NumberOfTableDimensions=3  BreakpointsForDimension1=Alpha  BreakpointsForDimension2=Vinf  BreakpointsForDimension3=Vh  BeginIndexSearchUsingPreviousIndexResult=on  Table=ToverTh  InterpMethod=Cubic spline  InputSameDT=on
  thrust_multiplier : Outport  OutDataType=sfix(16)  OutScaling=2^0
  wires:
  Saturation/1 -> Divide/2
  Demux/3 -> Unary Minus/1
  Unary Minus/1 -> Divide/1
  Abs/1 -> Switch/2
  Constant/1 -> Switch/1
  v_i Lookup Table (n-D)/1 -> Switch/3
  Switch/1 -> Saturation1/1
  Trigonometric Function/1 -> v_i Lookup Table (n-D)/1, Abs/1  "alpha"
  Divide/1 -> Trigonometric Function/1
  Demux/2 -> T1/1
  Demux/1 -> T/1
  Math Function/1 -> Saturation/1, v_i Lookup Table (n-D)/2  "v_inf"
  Dot Product/1 -> Math Function/1
  v_body_relative/1 -> Zero-Order Hold2/1
  motor_thrusts/1 -> Zero-Order Hold1/1
  Zero-Order Hold1/1 -> "v_h "/1
  Zero-Order Hold2/1 -> Demux/1, Dot Product/2, Dot Product/1
  Saturation1/1 -> Rate Transition/1
  "v_h "/1 -> v_i Lookup Table (n-D)/3  "v_h"
  Rate Transition/1 -> thrust_multiplier/1

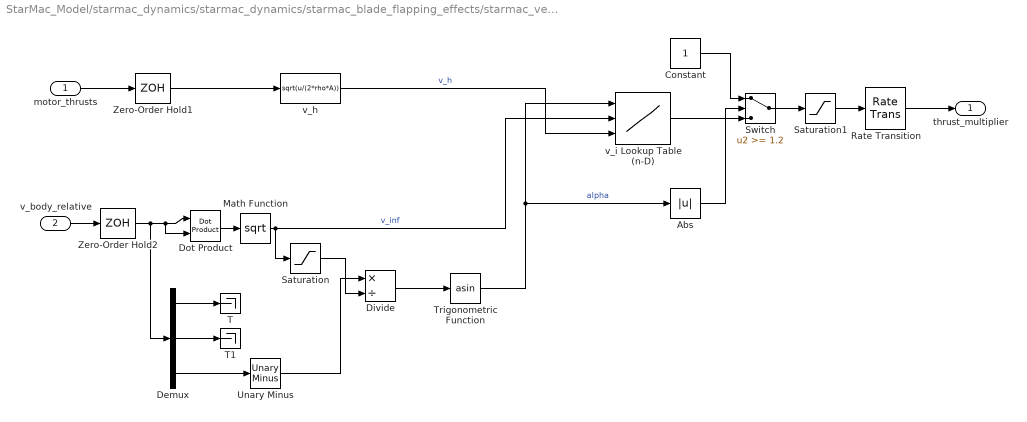
== system StarMac_Model/starmac_dynamics/starmac_dynamics/starmac_blade_flapping_effects/starmac_vertical_effect_dynamics/starmac_motor_vertical_effect_dynamics1 ==
  motor_thrusts : Inport  OutDataType=sfix(16)  OutScaling=2^0
  v_body_relative : Inport  Port=2  OutDataType=sfix(16)  OutScaling=2^0
  Abs : Abs
  Constant : Constant  OutDataType=sfix(16)  OutScaling=2^0
  Demux : Demux  Outputs=3
  Divide : Product  Inputs=*/  OutDataType=sfix(16)  OutScaling=2^-10
  Dot Product : simulink/Math Operations/Dot Product  InputSameDT=on  OutDataType=sfix(16)  OutScaling=2^-10  DoSatur=off
  Math Function : Math  Operator=sqrt  OutDataType=sfix(16)  OutScaling=2^0  SaturateOnIntegerOverflow=on
  Rate Transition : RateTransition
  Saturation : Saturate  UpperLimit=500000  LowerLimit=0.0000000001
  Saturation1 : Saturate  UpperLimit=2  LowerLimit=0.5
  Switch : Switch  Threshold=1.2
  T : Terminator
  T1 : Terminator
  Trigonometric Function : Trigonometry  Operator=asin
  Unary Minus : simulink/Math Operations/Unary Minus  DoSatur=off
  Zero-Order Hold1 : ZeroOrderHold  SampleTime=tau_motor
  Zero-Order Hold2 : ZeroOrderHold  SampleTime=tau_motor
  "v_h " : Fcn  Expr=sqrt(u/(2*rho*A))
  v_i Lookup Table (n-D) : Lookup_n-D  NumberOfTableDimensions=3  BreakpointsForDimension1=Alpha  BreakpointsForDimension2=Vinf  BreakpointsForDimension3=Vh  BeginIndexSearchUsingPreviousIndexResult=on  Table=ToverTh  InterpMethod=Cubic spline  InputSameDT=on
  thrust_multiplier : Outport  OutDataType=sfix(16)  OutScaling=2^0
  wires:
  Saturation/1 -> Divide/2
  Demux/3 -> Unary Minus/1
  Unary Minus/1 -> Divide/1
  Abs/1 -> Switch/2
  Constant/1 -> Switch/1
  v_i Lookup Table (n-D)/1 -> Switch/3
  Switch/1 -> Saturation1/1
  Trigonometric Function/1 -> v_i Lookup Table (n-D)/1, Abs/1  "alpha"
  Divide/1 -> Trigonometric Function/1
  Demux/2 -> T1/1
  Demux/1 -> T/1
  Math Function/1 -> Saturation/1, v_i Lookup Table (n-D)/2  "v_inf"
  Dot Product/1 -> Math Function/1
  v_body_relative/1 -> Zero-Order Hold2/1
  motor_thrusts/1 -> Zero-Order Hold1/1
  Zero-Order Hold1/1 -> "v_h "/1
  Zero-Order Hold2/1 -> Demux/1, Dot Product/2, Dot Product/1
  Saturation1/1 -> Rate Transition/1
  "v_h "/1 -> v_i Lookup Table (n-D)/3  "v_h"
  Rate Transition/1 -> thrust_multiplier/1

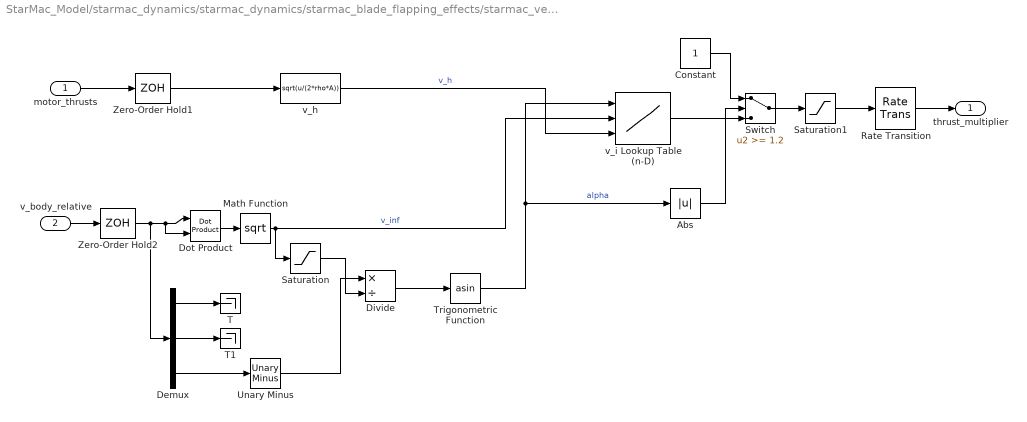
== system StarMac_Model/starmac_dynamics/starmac_dynamics/starmac_blade_flapping_effects/starmac_vertical_effect_dynamics/starmac_motor_vertical_effect_dynamics2 ==
  motor_thrusts : Inport  OutDataType=sfix(16)  OutScaling=2^0
  v_body_relative : Inport  Port=2  OutDataType=sfix(16)  OutScaling=2^0
  Abs : Abs
  Constant : Constant  OutDataType=sfix(16)  OutScaling=2^0
  Demux : Demux  Outputs=3
  Divide : Product  Inputs=*/  OutDataType=sfix(16)  OutScaling=2^-10
  Dot Product : simulink/Math Operations/Dot Product  InputSameDT=on  OutDataType=sfix(16)  OutScaling=2^-10  DoSatur=off
  Math Function : Math  Operator=sqrt  OutDataType=sfix(16)  OutScaling=2^0  SaturateOnIntegerOverflow=on
  Rate Transition : RateTransition
  Saturation : Saturate  UpperLimit=500000  LowerLimit=0.0000000001
  Saturation1 : Saturate  UpperLimit=2  LowerLimit=0.5
  Switch : Switch  Threshold=1.2
  T : Terminator
  T1 : Terminator
  Trigonometric Function : Trigonometry  Operator=asin
  Unary Minus : simulink/Math Operations/Unary Minus  DoSatur=off
  Zero-Order Hold1 : ZeroOrderHold  SampleTime=tau_motor
  Zero-Order Hold2 : ZeroOrderHold  SampleTime=tau_motor
  "v_h " : Fcn  Expr=sqrt(u/(2*rho*A))
  v_i Lookup Table (n-D) : Lookup_n-D  NumberOfTableDimensions=3  BreakpointsForDimension1=Alpha  BreakpointsForDimension2=Vinf  BreakpointsForDimension3=Vh  BeginIndexSearchUsingPreviousIndexResult=on  Table=ToverTh  InterpMethod=Cubic spline  InputSameDT=on
  thrust_multiplier : Outport  OutDataType=sfix(16)  OutScaling=2^0
  wires:
  Saturation/1 -> Divide/2
  Demux/3 -> Unary Minus/1
  Unary Minus/1 -> Divide/1
  Abs/1 -> Switch/2
  Constant/1 -> Switch/1
  v_i Lookup Table (n-D)/1 -> Switch/3
  Switch/1 -> Saturation1/1
  Trigonometric Function/1 -> v_i Lookup Table (n-D)/1, Abs/1  "alpha"
  Divide/1 -> Trigonometric Function/1
  Demux/2 -> T1/1
  Demux/1 -> T/1
  Math Function/1 -> Saturation/1, v_i Lookup Table (n-D)/2  "v_inf"
  Dot Product/1 -> Math Function/1
  v_body_relative/1 -> Zero-Order Hold2/1
  motor_thrusts/1 -> Zero-Order Hold1/1
  Zero-Order Hold1/1 -> "v_h "/1
  Zero-Order Hold2/1 -> Demux/1, Dot Product/2, Dot Product/1
  Saturation1/1 -> Rate Transition/1
  "v_h "/1 -> v_i Lookup Table (n-D)/3  "v_h"
  Rate Transition/1 -> thrust_multiplier/1

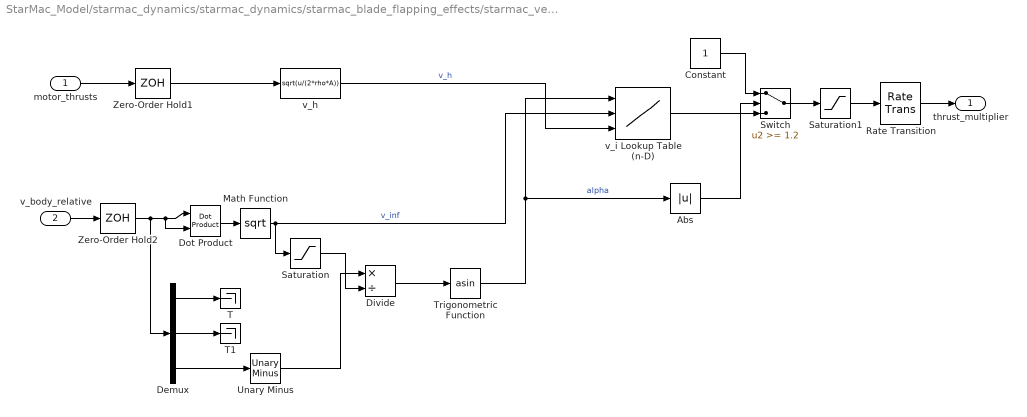
== system StarMac_Model/starmac_dynamics/starmac_dynamics/starmac_blade_flapping_effects/starmac_vertical_effect_dynamics/starmac_motor_vertical_effect_dynamics3 ==
  motor_thrusts : Inport  OutDataType=sfix(16)  OutScaling=2^0
  v_body_relative : Inport  Port=2  OutDataType=sfix(16)  OutScaling=2^0
  Abs : Abs
  Constant : Constant  OutDataType=sfix(16)  OutScaling=2^0
  Demux : Demux  Outputs=3
  Divide : Product  Inputs=*/  OutDataType=sfix(16)  OutScaling=2^-10
  Dot Product : simulink/Math Operations/Dot Product  InputSameDT=on  OutDataType=sfix(16)  OutScaling=2^-10  DoSatur=off
  Math Function : Math  Operator=sqrt  OutDataType=sfix(16)  OutScaling=2^0  SaturateOnIntegerOverflow=on
  Rate Transition : RateTransition
  Saturation : Saturate  UpperLimit=500000  LowerLimit=0.0000000001
  Saturation1 : Saturate  UpperLimit=2  LowerLimit=0.5
  Switch : Switch  Threshold=1.2
  T : Terminator
  T1 : Terminator
  Trigonometric Function : Trigonometry  Operator=asin
  Unary Minus : simulink/Math Operations/Unary Minus  DoSatur=off
  Zero-Order Hold1 : ZeroOrderHold  SampleTime=tau_motor
  Zero-Order Hold2 : ZeroOrderHold  SampleTime=tau_motor
  "v_h " : Fcn  Expr=sqrt(u/(2*rho*A))
  v_i Lookup Table (n-D) : Lookup_n-D  NumberOfTableDimensions=3  BreakpointsForDimension1=Alpha  BreakpointsForDimension2=Vinf  BreakpointsForDimension3=Vh  BeginIndexSearchUsingPreviousIndexResult=on  Table=ToverTh  InterpMethod=Cubic spline  InputSameDT=on
  thrust_multiplier : Outport  OutDataType=sfix(16)  OutScaling=2^0
  wires:
  Saturation/1 -> Divide/2
  Demux/3 -> Unary Minus/1
  Unary Minus/1 -> Divide/1
  Abs/1 -> Switch/2
  Constant/1 -> Switch/1
  v_i Lookup Table (n-D)/1 -> Switch/3
  Switch/1 -> Saturation1/1
  Trigonometric Function/1 -> v_i Lookup Table (n-D)/1, Abs/1  "alpha"
  Divide/1 -> Trigonometric Function/1
  Demux/2 -> T1/1
  Demux/1 -> T/1
  Math Function/1 -> Saturation/1, v_i Lookup Table (n-D)/2  "v_inf"
  Dot Product/1 -> Math Function/1
  v_body_relative/1 -> Zero-Order Hold2/1
  motor_thrusts/1 -> Zero-Order Hold1/1
  Zero-Order Hold1/1 -> "v_h "/1
  Zero-Order Hold2/1 -> Demux/1, Dot Product/2, Dot Product/1
  Saturation1/1 -> Rate Transition/1
  "v_h "/1 -> v_i Lookup Table (n-D)/3  "v_h"
  Rate Transition/1 -> thrust_multiplier/1
